simulink model "simulink_model_compare"  (R2016b)
settings: Solver=VariableStepAuto  StartTime=0.0  StopTime=1  RelTol=1e-3
values from neighbouring files (symbols this model uses):
  linsys = lin_sys(m,M,l,g,b,k)    [main.m]
  linsys_init = z0    [main.m]
  z0 = [theta_rad_init; 0; 0; 0]    [main.m]
settings Model: Creator=pluspole  LastModifiedBy=pluspole

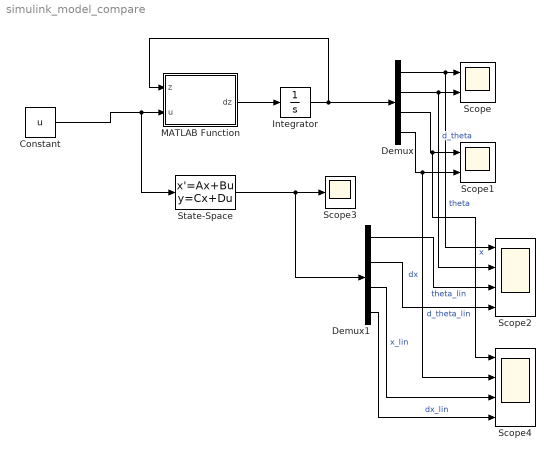
== system simulink_model_compare ==
  Constant : Constant  Value=u
  Demux : Demux
  Demux1 : Demux
  Integrator : Integrator  InitialCondition=z0
  MATLAB Function : MATLAB Function  TreatAsAtomicUnit=on
  Scope : Scope  NumInputPorts=2
  Scope1 : Scope  NumInputPorts=2
  Scope2 : Scope  NumInputPorts=4
  Scope3 : Scope
  Scope4 : Scope  NumInputPorts=4
  State-Space : StateSpace  A=linsys.A  B=linsys.B  C=linsys.C  D=linsys.D  X0=linsys_init
  wires:
  MATLAB Function/1(dz) -> Integrator/1
  Integrator/1 -> Demux/1, MATLAB Function/1(z)
  Constant/1 -> State-Space/1, MATLAB Function/2(u)
  Demux/1 -> Scope2/1, Scope/1  "theta"
  Demux/2 -> Scope2/2, Scope/2  "d_theta"
  Demux/3 -> Scope4/1, Scope1/1  "x"
  Demux/4 -> Scope4/2, Scope1/2  "dx"
  State-Space/1 -> Scope3/1, Demux1/1
  Demux1/1 -> Scope2/3  "theta_lin"
  Demux1/2 -> Scope2/4  "d_theta_lin"
  Demux1/3 -> Scope4/3  "x_lin"
  Demux1/4 -> Scope4/4  "dx_lin"

== matlab function simulink_model_compare/MATLAB Function ==
  data: z input; u input; dz output; p parameter
function dz = fcn(z,u, p)

m=p.m;
M=p.M;
l=p.l;
g=p.g;
b=p.b;
k=p.k;

c1=cos(z(1));
s1=sin(z(1));

dz=zeros(4,1);

dz(1,1) = z(2);

dz(2,1) = ((u*c1)-(b*z(3)*c1)-((M+m)*g*s1)+(m*l*c1*s1*(z(2)^2))+((M+m)*((k*z(2))/(l*m))) )/(m*l*(c1^2)-((M+m)*l));
%dy(4,1) = (1/D)*((m+M)*m*g*L*Sy - m*L*Cy*(m*L*y(4)^2*Sy - d*y(2))) - m*L*Cy*(1/D)*u +.01*randn;

dz(3,1) = z(4);

dz(4,1) = (u-(b*z(3))+(m*l*s1*(z(2)^2))-(m*g*c1*s1)+(c1*(k/l)*z(2)))/((M+m)-(m*(c1^2)));
%dy(2,1) = (1/D)*(-m^2*L^2*g*Cy*Sy + m*L^2*(m*L*y(4)^2*Sy - d*y(2))) + m*L*L*(1/D)*u;
